simulink model "untitled1"  (R2020a)
settings: Solver=VariableStepAuto  StartTime=0.0  StopTime=10.0  RelTol=1e-3
values from neighbouring files (symbols this model uses):
  A = [2,3;-1,4]    [Initialize.m]
  B = [0;1]    [Initialize.m]
  C = [1,0]    [Initialize.m]
  G = -inv(C*inv(A-B*K)*B)    [Initialize.m]
  K = lqr(A,B,Q,R)    [Initialize.m]
settings Model: Creator=prans  LastModifiedBy=prans

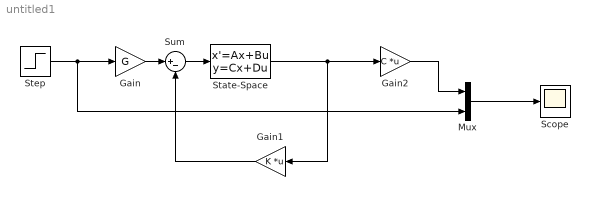
== system untitled1 ==
  Gain : Gain  Gain=G
  Gain1 : Gain  Gain=K  Multiplication=Matrix(K*u)
  Gain2 : Gain  Gain=C  Multiplication=Matrix(K*u)
  Mux : Mux  Inputs=2
  Scope : Scope
  State-Space : StateSpace  A=A  B=B  C=eye(2)  D=[0;0]  InitialCondition=0
  Step : Step  SampleTime=0
  Sum : Sum  Inputs=|+-
  wires:
  Step/1 -> Mux/2, Gain/1
  Gain/1 -> Sum/1
  Sum/1 -> State-Space/1
  Gain1/1 -> Sum/2
  State-Space/1 -> Gain1/1, Gain2/1
  Gain2/1 -> Mux/1
  Mux/1 -> Scope/1
